simulink model "Copy_of_MPC_control"  (R2018a)
settings: Solver=FixedStepAuto  StartTime=0  StopTime=Tend  FixedStep=0.001  RelTol=5e-3
model workspace (MAT data in the model file):
  A_mu = 10
  B_reff = 8.386
  Cz = 7766.25
  DCT_Param.Transmission.Ratios = [3.78 2.18 1.43 1.03 0.935 0.84]
  DCT_Param.Transmission.Shaft_Inertia_Odd = 0.0023
  DCT_Param.Transmission.Shaft_Inertia_Even = 0.0009
  DCT_Param.Transmission.Shaft_Inertia_Output = 0.008
  DCT_Param.Transmission.Gear_Inertia = 0.001
  DCT_Param.Transmission.Gear_Efficiency = 0.94
  DCT_Param.Transmission.Gear_Ang_Vel_Thr = 0.01
  DCT_Param.Transmission.Shaft_Velocity_Odd = 0
  DCT_Param.Transmission.Shaft_Velocity_Even = 0
  DCT_Param.Transmission.Shaft_Velocity_Output = 0
  DCT_Param.Transmission.Gear_Initial_Velocity = 0
  DCT_Param.Transmission.Abstract.Compliance = 100000
  DCT_Param.Transmission.Abstract.Damping = 10000
  DCT_Param.Transmission.Abstract.Ratio_Time_Const = 0.05
  DCT_Param.Transmission.Abstract.Shift_Gear_Delay = 25
  DCT_Param.Clutch.Torque_Radius = 130
  DCT_Param.Clutch.Num_Friction_Surfaces = 4
  DCT_Param.Clutch.Engagement_Piston_Area = 0.001
  DCT_Param.Clutch.Kinetic_Friction_Coeff = 0.3
  DCT_Param.Clutch.Static_Friction_Coeff = 0.31
  DCT_Param.Clutch.Derating_Factor = 1
  DCT_Param.Clutch.Clutch_Velocity_Tolerance = 0.001
  DCT_Param.Clutch.Threshold_Pressure = 1
  DCT_Param.Clutch.Drag_Torque_Coeff = 0
  DCT_Param.Dog_Clutch.Max_Torque = 1000
  DCT_Param.Dog_Clutch.Teeth_Mean_Radius = 50
  DCT_Param.Dog_Clutch.Tooth_Height = 10
  DCT_Param.Dog_Clutch.Ring_Hub_Clearance = 3
  DCT_Param.Dog_Clutch.Ring_Stop_Stiffness = 1000000
  DCT_Param.Dog_Clutch.Ring_Stop_Damping = 1000
  DCT_Param.Dog_Clutch.Shift_Linkage_Damping = 100
  DCT_Param.Dog_Clutch.Max_Engage_Velocity = 1000000
  DCT_Param.Dog_Clutch.Tooth_Engage_Overlap = 3
  DCT_Param.Vehicle.Mass = 1600
  DCT_Param.Vehicle.Wheels_Per_Axle = 2
  DCT_Param.Vehicle.Distance_CG_FrontAxle = 1.7
  DCT_Param.Vehicle.Distance_CG_RearAxle = 2
  DCT_Param.Vehicle.Distance_CG_Ground = 0.5
  DCT_Param.Vehicle.Frontal_Area = 3
  DCT_Param.Vehicle.Aero_Drag_Coeff = 0.4
  DCT_Param.Vehicle.Initial_Velocity = 0
  DCT_Param.Vehicle.Final_Drive_Ratio = 3.7
  DCT_Param.Vehicle.Final_Drive_Efficiency = 0.86
  DCT_Param.Vehicle.Final_Drive_Vel_Thresh = 0.01
  DCT_Param.Vehicle.Side_Shaft_Inertia = 0.01
  DCT_Param.Vehicle.Side_Shaft_Initial_Velocity = 0
  DCT_Param.Vehicle.Tire.Radius = 0.312
  DCT_Param.Vehicle.Tire.Inertia = 0.5
  DCT_Param.Vehicle.Tire.Initial_Velocity = 0
  DCT_Param.Vehicle.Tire.Slip_Vel_Thresh = 0.1
  DCT_Param.Vehicle.Tire.Nominal_Vertical_Load = 4000
  DCT_Param.Vehicle.Tire.C_Coeff = 1.685
  DCT_Param.Vehicle.Tire.D_Coeff = [1.21 -0.037]
  DCT_Param.Vehicle.Tire.E_Coeff = [0.344 0.095 -0.02 0]
  DCT_Param.Vehicle.Tire.BCD_Coeff = [21.51 -0.163 0.245]
  DCT_Param.Vehicle.Tire.H_Coeff = [-0.002 0.002]
  DCT_Param.Vehicle.Tire.V_Coeff = [0 0]
  DCT_Param.ICE.Max_Power = 100000
  DCT_Param.ICE.Speed_At_Max_Power = 5500
  DCT_Param.ICE.Max_Speed = 7000
  DCT_Param.ICE.Stall_Speed = 200
  DCT_Param.ICE.Shaft_Inertia = 0.2
  DCT_Param.ICE.Initial_Velocity = 800
  DCT_Param.ICE.Idle_Ref_Spd = 800
  DCT_Param.ICE.Engine_Time_Constant = 0.2
  DCT_Param.ICE.Initial_Normalized_Throttle = 0
  DCT_Param.ICE.Speed_Threshold = 20
  DCT_Param.ICE.FC.Speed_Vector = [0 368.421052632 736.842105263 1105.26315789 1473.68421053 1842.10526316 2210.52631579 2578.94736842 2947.36842105 3315.78947368 3684.21052632 4052.63157895 4421.05263158 4789.47368421 5157.89473684 5526.31578947 5894.73684211 6263.15789474 6631.57894737 7000]
  DCT_Param.ICE.FC.Torque_Vector = [0 10.5263157895 21.0526315789 31.5789473684 42.1052631579 52.6315789474 63.1578947368 73.6842105263 84.2105263158 94.7368421053 105.263157895 115.789473684 126.315789474 136.842105263 147.368421053 157.894736842 168.421052632 178.947368421 189.473684211 200]
  DCT_Param.ICE.FC.Consumption_Table = [0.262945178015 0.225304787522 0.201465019624 0.191425874321 0.195187351614 0.212749451502 0.244112173984 0.289275519063 0.348239486736 0.421004077004 0.507569289868 0.607935125326 ... (400 elements, 20x20)]
  DCT_Param.Shift_Map_Example.Pedal_Positions = [0.1 0.4 0.5 0.9]
  DCT_Param.Shift_Map_Example.Upshift_Speeds = [11  20  26  34.5  43; 14  26  35  44.5  55; 17  31  42  52.5  65; 21  39  52  66.5  80]
  DCT_Param.Shift_Map_Example.Downshift_Speeds = [8.9  17  23.6  32.4  40.8; 11.5  22.7  32  41.6  52.2; 14  27  38.1  50  62; 18  33  48  62.6  76.2]
  DCT_Param.Shift_Map_ORIG.Pedal_Positions = [0.1 0.4 0.5 0.9]
  DCT_Param.Shift_Map_ORIG.Upshift_Speeds = [11.5  23.5  35.5  45.5  55.5; 14.5  26.5  38.5  48.5  58.5; 17.5  29.5  41.5  51.5  61.5; 20.5  32.5  44.5  54.5  64.5]
  DCT_Param.Shift_Map_ORIG.Downshift_Speeds = [8.5  20.5  32.5  42.5  52.5; 11.5  23.5  35.5  45.5  55.5; 14.5  26.5  38.5  48.5  58.5; 17.5  29.5  41.5  51.5  61.5]
  DCT_Param.Shift_Map_OPT.Pedal_Positions = [0.1 0.4 0.5 0.9]
  DCT_Param.Shift_Map_OPT.Upshift_Speeds = [17.8469  29.8469  35.8159  41.2981  46.3004; 19.2469  33.9778  43.9778  53.9778  63.9778; 24.5469  41.9778  62.1778  78.5778  106.9778; 27.5469  59.3778  99.0445  109.0445  119.0445]
  DCT_Param.Shift_Map_OPT.Downshift_Speeds = [14.8469  26.8469  32.8159  38.2981  43.3004; 16.2469  30.9778  40.9778  50.9778  60.9778; 21.5469  38.9778  59.1778  75.5778  103.9778; 24.5469  56.3778  96.0445  106.0445  116.0445]
  DCT_Param.Shift_Map.Pedal_Positions = [0.1 0.4 0.5 0.9]
  DCT_Param.Shift_Map.Upshift_Speeds = [11.5  23.5  35.5  45.5  55.5; 14.5  26.5  38.5  48.5  58.5; 17.5  29.5  41.5  51.5  61.5; 20.5  32.5  44.5  54.5  64.5]
  DCT_Param.Shift_Map.Downshift_Speeds = [8.5  20.5  32.5  42.5  52.5; 11.5  23.5  35.5  45.5  55.5; 14.5  26.5  38.5  48.5  58.5; 17.5  29.5  41.5  51.5  61.5]
  DCT_Param.Control.Clutch.Min_Lock_Pressure = 2000000
  DCT_Param.Control.Clutch.Max_Lock_Pressure = 5000000
  DCT_Param.Control.Clutch.Max_Unlock_Pressure = 500000
  DCT_Param.Control.Engine_Start_RPM = 800
  DCT_Param.Control.Engine_Stop_RPM = 790
  DCT_Param.Control.Mode_Logic_TS = 0.1
  DCT_Param.Control.ICE.Kp = 0.02
  DCT_Param.Control.ICE.Ki = 0.01
  DCT_Param.Control.Gen.Kp = 10
  DCT_Param.Control.Gen.Ki = 3
  DCT_Param.Control.Mot.Kp = 500
  DCT_Param.Control.Mot.Ki = 300
  DCT_Param.Control.Veh_Spd.Kp = 0.02
  DCT_Param.Control.Veh_Spd.Ki = 0.04
  DCT_Param.Driver.Kp = 400
  DCT_Param.Driver.Ki = 0.001
  DCT_Param.Driver.Pedal_Filter_Const = 0.01
  DCT_Param.Dog_Clutches.Pulse_Delay = 50
  DCT_Param.Dog_Clutches.Pulse_Length = 20
  DCT_Param.Animation.Teeth_Ratios = [0.338461538462 0.555555555556 0.916666666667 0.96 1.17948717949 1.92307692308]
  DCT_Param.Animation.Teeth_Ratios_Reverse = [0.458333333333 0.75]
  DCT_Param.Shift_Map_OPT506.Pedal_Positions = [0.1 0.4 0.5 0.9]
  DCT_Param.Shift_Map_OPT506.Upshift_Speeds = [18  30.2  48.3  67.3322  77.3429; 20.1  36.85  66.6178  76.7537  86.7537; 21.1  40.25  71.0189  81.0189  91.7873; 24.1  63.75  80.7523  105.9489  115.9489]
  DCT_Param.Shift_Map_OPT506.Downshift_Speeds = [15  27.2  45.3  64.3322  74.3429; 17.1  33.85  63.6178  73.7537  83.7537; 18.1  37.25  68.0189  78.0189  88.7873; 21.1  60.75  77.7523  102.9489  112.9489]
  DCT_Param.Shift_Map_OPTAbsRea176.Pedal_Positions = [0.1 0.4 0.5 0.9]
  DCT_Param.Shift_Map_OPTAbsRea176.Upshift_Speeds = [17.8469  29.8469  35.7875  44.0901  49.4243; 18.9219  34.1312  45.8256  59.7585  69.7585; 32.1719  43.4585  53.51  103.2151  114.6401; 35.1719  59.2585  99.5217  109.5217  119.5217]
  DCT_Param.Shift_Map_OPTAbsRea176.Downshift_Speeds = [14.8469  26.8469  32.7875  41.0901  46.4243; 15.9219  31.1312  42.8256  56.7585  66.7585; 29.1719  40.4585  50.51  100.2151  111.6401; 32.1719  56.2585  96.5217  106.5217  116.5217]
  D_reff = 0.25826
  Downshift_Speeds = [9.5625  23.0625  36.5625  47.8125  59.0625  68.90625  78.75; 12.9375  26.4375  39.9375  51.1875  62.4375  72.84375  83.25; 16.3125  29.8125  43.3125  54.5625  65.8125  76.78125  87.75; 19.6875  33.1875  46.6875  57.9375  69.1875  80.71875  92.25]
  Pedal_Positions = [0.1 0.4 0.5 0.9]
  SUS.Stiffness = 24000
  SUS.Damping.Constant = 1262
  SUS.Damping.Rebound = [4040 4950 2883 2043]
  SUS.Damping.Compression = [3600 3420 1863 1472]
  SUS.PistonSpeed = [0.05 0.1 0.3 0.6]
  SUS.UnsprungMass.Fr = 21.0693333333
  SUS.UnsprungMass.Rr = 21.0693333333
  Upshift_Speeds = [12.9375  26.4375  39.9375  51.1875  62.4375  72.84375  83.25; 16.3125  29.8125  43.3125  54.5625  65.8125  76.78125  87.75; 19.6875  33.1875  46.6875  57.9375  69.1875  80.71875  92.25; 33  52.5  77.25  100.5  138.75  161.875  185]
  VEH.Mass = 1181
  VEH.StaticNormalFrontLoad.FR = 264.666666667
  VEH.StaticNormalFrontLoad.FL = 264.666666667
  VEH.StaticNormalRearLoad.RR = 322
  VEH.StaticNormalRearLoad.RL = 322
  VEH.WheelBase = 3.075
  VEH.FrontAxlePositionfromCG = 1.515
  VEH.RearAxlePositionfromCG = 1.504
  VEH.HeightCG = 0.134
  VEH.FrontalArea = 2.11
  VEH.DragCoefficient = 0.33
  VEH.NumberOfWheelsPerAxle = 2
  VEH.Thread.FR = 1.705
  VEH.Thread.RR = 1.705
  VEH.PitchMomentInertia = 1922.66666667
  VEH.RollMomentInertia = 432.333333333
  VEH.YawMomentInertia = 2066
  VEH.SteeringRatio = 18
  VEH.TrackWidth = 1.922
  VEH.SprungMass = 1096.72266667
  VEH.InitialLongPosition = 0
  VEH.InitialLatPosition = 3.125
  VEH.InitialVertPosition = 0.0111
  VEH.InitialRollAngle = 0
  VEH.InitialPitchAngle = -0.000732
  VEH.InitialYawAngle = 0
  VEH.InitialLongVel = 0
  VEH.InitialLatVel = 0
  VEH.InitialVertVel = 0
  VEH.InitialRollRate = 0
  VEH.InitialPitchRate = 0
  VEH.InitialYawRate = 0
  V_o = 16.7
  V_xlow = 1
  WH.Tire.Radius.Front = 0.384
  WH.Tire.Radius.Rear = 0.401
  WH.Tire.Sidewall = 0.245
  WH.Tire.RollingResistCoeff = 0.0103
  WH.Tire.Magic.B = 10
  WH.Tire.Magic.C = 1.9
  WH.Tire.Magic.D = 1
  WH.Tire.Magic.E = 0.97
  WH.Tire.Magic.Bx = 12
  WH.Tire.Magic.Cx = 1.9
  WH.Tire.Magic.Dx = 0.72
  WH.Tire.Magic.Ex = 0.95
  WH.Tire.Magic.By = 12
  WH.Tire.Magic.Cy = 1.3
  WH.Tire.Magic.Dy = 0.75
  WH.Tire.Magic.Ey = 0.2
  WH.Tire.Front.Ky = 40000
  WH.Tire.Rear.Ky = 40000
  WH.Tire.Kz = 320000
  WH.Tire.Damping = 100
  WH.Inertia = 1.00333333333
  WH.Mass = 11.4333333333
  WH.DampingCoefficient = 0.01
  WH.VelocityTol = 0.1
  a = 1.4
  alpha_max = 1.5
  alpha_min = -1.5
  b = 1.8
  c_zo = 209651
  epsilon = 0.1
  h = 0.134
  path.ISO3888p2.x = [0 2 12 25.5 36.5 49 61]
  path.ISO3888p2.y = [0 0 0 3.725 3.725 0 0]
  path.ISO3888p2.ylb = [1.225 1.225 1.225 4.725 4.725 1.5 1.5]
  path.ISO3888p2.yrb = [-1.225 -1.225 -1.225 2.225 2.225 -1.5 -1.5]
  path.CUSC.x = [10.668 21.336 36.576 54.864 73.152]
  path.CUSC.y = [0 0 5.1816 0 0]
  path.CUSC.ylb = [1.2192 1.2192 7.0104 1.8288 1.8288]
  path.CUSC.yrb = [-1.2192 -1.2192 3.3528 -1.8288 -1.8288]
  pio = 220000
  q_Fcx = 0
  q_Fz2 = 15.4
  q_Fzy = 0
  q_reo = 0.9974
  q_sx1 = -0.007764
  q_sx10 = 0.2824
  q_sx11 = 5.349
  q_sx12 = 0
  q_sx13 = 0
  q_sx14 = 0
  q_sx2 = 1.1915
  q_sx3 = 0.013948
  q_sx4 = 4.912
  q_sx5 = 1.02
  q_sx6 = 22.83
  q_sx7 = 0.7104
  q_sx8 = -0.023393
  q_sx9 = 0.6581
  q_sy1 = 0.00702
  q_sy2 = 0
  q_sy3 = 0.001515
  q_sy4 = 8.514e-05
  q_sy5 = 0
  q_sy6 = 0
  q_sy7 = 0.9008
  q_sy8 = -0.4089
  q_v1 = 0.0007742
  q_v2 = 0.04667
  r_Bx1 = 12.531
  r_Bx2 = 9.532
  r_Bx3 = 0
  r_By1 = 10.615
  r_By2 = 7.705
  r_By3 = 3.433e-06
  r_By4 = 0
  r_Cx1 = 1.019
  r_Cy1 = 1.0585
  r_Ex1 = -0.4487
  r_Ex2 = -0.4726
  r_Ey1 = 0.3132
  r_Ey2 = 7.63e-06
  r_Hx1 = 0.0002374
  r_Hy1 = 0.011646
  r_Hy2 = 7.63e-06
  r_Vy1 = 0.05654
  r_Vy2 = 7.63e-06
  r_Vy3 = 0
  r_Vy4 = 99.9
  r_Vy5 = 2
  r_Vy6 = 15.814
  r_o = 0.3135
  vehWidth = 2
  w = 1
undefined symbols (not defined in the file): C_Brake, C_Final, C_Front, C_Front_1, C_Front_2, C_Middle, C_out_Brake, C_out_Final, C_out_Front, C_out_Front_1, C_out_Front_2, C_out_Middle, Co, Cok_Brake, Cok_Final, Cok_Front_1, Cok_Front_2, Cok_Middle, Cso, D_out_Brake, D_out_Final, D_out_Front, D_out_Front_1, D_out_Front_2, D_out_Middle, Earlytochange, Earlytochange2, F, F_Brake, F_Final, F_Front, F_Front_1, F_Front_2, F_Middle, Fs, G_Brake, G_Final, G_Front_1, G_Front_2, G_Middle, G_sys_Brake, G_sys_Final, G_sys_Front, G_sys_Front_1, G_sys_Front_2, G_sys_Middle, Gd, Gd_Brake, Gd_Final, Gd_Front, Gd_Front_1, Gd_Front_2, Gd_Middle, Go, Gsd, Gso, H_Brake, H_Final, H_Front_1, H_Front_2 ... (+60)
libraries: simulink x10, sim3dlib x4, autolibutils x2, vehdynlibviscommon x2
(part 1 of 8)
settings Model: ModifiedByFormat=The MathWorks, Inc.  Creator=The MathWorks, Inc.  LastModifiedBy=The MathWorks, Inc.
settings SolverCC: ZeroCrossAlgorithm=Adaptive  DecoupledContinuousIntegration=on  MinimalZcImpactIntegration=on
settings DebuggingCC: SignalInfNanChecking=error  ArtificialAlgebraicLoopMsg=none  IgnoredZcDiagnostic=none  ModelReferenceExtraNoncontSigs=none
settings ModelReferenceCC: UpdateModelReferenceTargets=IfOutOfDate  EnableParallelModelReferenceBuilds=on  ModelReferenceMinAlgLoopOccurrences=on  PropagateSignalLabelsOutOfModel=off
settings RTWCC: BuildConfiguration=Faster Runs

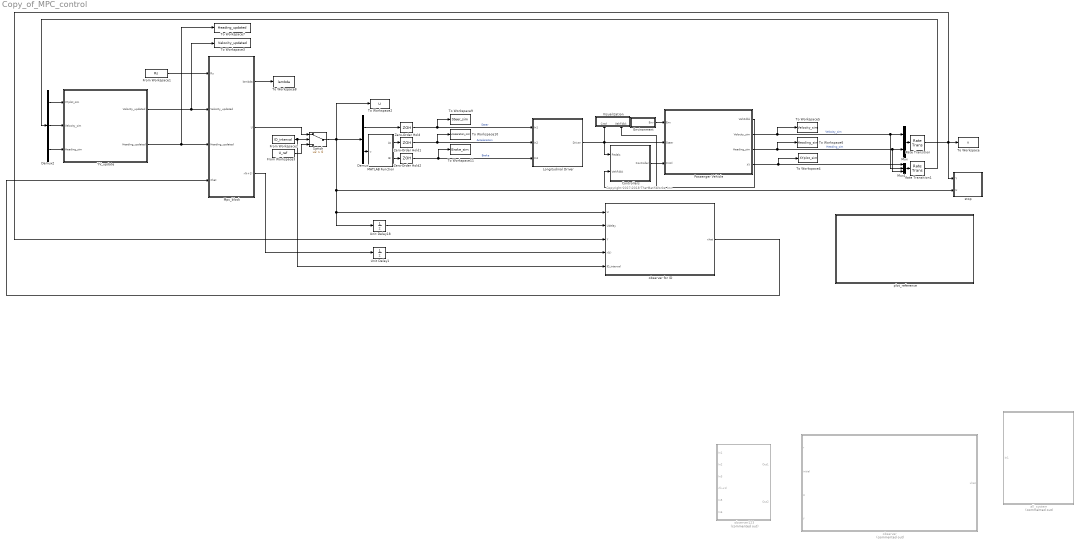
== system Copy_of_MPC_control ==
  note: Copyright 2017-2018 The MathWorks, Inc.
  Controllers : Subsystem
      mask Display: image('SystemControllers.png')
  Demux : Demux  Outputs=2
  Demux2 : Demux  Outputs=3
  Environment : Subsystem  TreatAsAtomicUnit=on
      mask Display: disp('Environment')
  From Workspace1 : FromWorkspace  VariableName=Rs  SampleTime=Ts
  From Workspace2 : FromWorkspace  VariableName=ID_interval  SampleTime=Ts
  From Workspace3 : FromWorkspace  VariableName=U_ref  SampleTime=Ts
  Longitudinal Driver : Subsystem  SystemSampleTime=Tf  VariantControl=0
      mask Display: image('longitudinal_driver_pedals.png');
  MATLAB Function : MATLAB Function  TreatAsAtomicUnit=on  SystemSampleTime=Ts
  Mpc_block : Subsystem  TreatAsAtomicUnit=on  SystemSampleTime=Ts
  Mux : Mux  Inputs=2
  Mux1 : Mux  Inputs=3
  Passenger Vehicle : Subsystem  TreatAsAtomicUnit=on
      settings: MinAlgLoopOccurrences=on
      mask Display: image('PassengerVehicle.png')
  Rate Transition : RateTransition  OutPortSampleTime=Ts
  Rate Transition1 : RateTransition  OutPortSampleTime=Ts
  Switch : Switch  Criteria=u2 > Threshold
  To Workspace : ToWorkspace  VariableName=Y  SampleTime=Ts
  To Workspace10 : ToWorkspace  VariableName=Acceleration_sim  SampleTime=Tf
  To Workspace11 : ToWorkspace  VariableName=Brake_sim  SampleTime=Tf
  To Workspace2 : ToWorkspace  VariableName=U  SampleTime=Ts
  To Workspace3 : ToWorkspace  VariableName=Velocity_updated  SampleTime=Ts
      settings: Save2DSignal=2-D array (concatenate along first dimension)
  To Workspace4 : ToWorkspace  VariableName=XYplot_sim  SampleTime=Ts
  To Workspace5 : ToWorkspace  VariableName=Velocity_sim  SampleTime=Ts
  To Workspace6 : ToWorkspace  VariableName=Heading_sim  SampleTime=Ts
  To Workspace7 : ToWorkspace  VariableName=Heading_updated  SampleTime=Ts
      settings: Save2DSignal=2-D array (concatenate along first dimension)
  To Workspace8 : ToWorkspace  VariableName=lambda  SampleTime=Ts
  To Workspace9 : ToWorkspace  VariableName=Steer_sim  SampleTime=-1
  Unit Delay1 : UnitDelay  InitialCondition=ro  SampleTime=Ts
  Unit Delay18 : UnitDelay  InitialCondition=[0;0]  SampleTime=Ts
  Visualization : Subsystem  TreatAsAtomicUnit=on
      mask Display: disp('Visualization')
  YV_update : Subsystem  TreatAsAtomicUnit=on
  Zero-Order Hold : ZeroOrderHold  SampleTime=Tf
  Zero-Order Hold1 : ZeroOrderHold  SampleTime=Tf
  Zero-Order Hold2 : ZeroOrderHold  SampleTime=Tf
  all_system : Subsystem  Commented=on
  observer : Subsystem  Commented=on
  observer for ID : Subsystem
  observer123 : Subsystem  Commented=on
  plot_reference : Subsystem
      settings: MinAlgLoopOccurrences=on
  stop : Subsystem
  wires:
  Longitudinal Driver/1(Driver) -> Passenger Vehicle/2(Steer), Controllers/1(Pedals), Visualization/1(Cntrl)
  Environment/1(Env) -> Passenger Vehicle/1(Env)
  Controllers/1(Controller) -> Passenger Vehicle/3(Cntrl)
  Passenger Vehicle/1(VehFdbk) -> Controllers/2(VehFdbk), Visualization/2(VehFdbk)
  Demux/1 -> Zero-Order Hold/1
  MATLAB Function/1(Ac) -> Zero-Order Hold1/1
  MATLAB Function/2(Br) -> Zero-Order Hold2/1
  Passenger Vehicle/3(Heading_sim) -> To Workspace6/1, Mux/2, Mux1/3  "Heading_sim"
  Mux/1 -> Rate Transition/1
  Demux/2 -> MATLAB Function/1(u)
  Zero-Order Hold/1 -> To Workspace9/1, Longitudinal Driver/1(In1)  "Steer"
  Zero-Order Hold1/1 -> To Workspace10/1, Longitudinal Driver/2(In2)  "Acceleration"
  Zero-Order Hold2/1 -> To Workspace11/1, Longitudinal Driver/3(In3)  "Brake"
  Passenger Vehicle/2(Velocity_sim) -> To Workspace5/1, Mux/1, Mux1/2  "Velocity_sim"
  YV_update/2(Heading_updated) -> Mpc_block/3(Heading_updated), To Workspace7/1
  YV_update/1(Velocity_updated) -> Mpc_block/2(Velocity_updated), To Workspace3/1
  Demux2/2 -> YV_update/2(Velocity_sim)
  Mux1/1 -> Rate Transition1/1
  Demux2/1 -> YV_update/1(XYplot_sim)
  Demux2/3 -> YV_update/3(Heading_sim)
  Rate Transition1/1 -> Demux2/1
  From Workspace1/1 -> Mpc_block/1(Rs)
  Passenger Vehicle/4(XY) -> To Workspace4/1, Mux1/1
  observer for ID/1(xhat) -> Mpc_block/4(Xhat)
  Rate Transition/1 -> observer for ID/3(Y), To Workspace/1, stop/1(Y)
  Mpc_block/3(r(k+1)) -> Unit Delay1/1
  Mpc_block/1(lambda) -> To Workspace8/1
  From Workspace2/1 -> observer for ID/5(ID_interval), Switch/2
  Mpc_block/2(U) -> Switch/1
  Switch/1 -> Demux/1, Unit Delay18/1, observer for ID/1(U), stop/2(U), To Workspace2/1
  From Workspace3/1 -> Switch/3
  Unit Delay18/1 -> observer for ID/2(Udelay)
  Unit Delay1/1 -> observer for ID/4(r(k))

== system Copy_of_MPC_control/Controllers ==
  Pedals : Inport
  VehFdbk : Inport  Port=2
  Brake Controller : Subsystem
  Bus Creator : BusCreator  Inputs=1
  Bus Creator1 : BusCreator  Inputs=1
  Bus Creator2 : BusCreator  Inputs=1
  Bus Creator3 : BusCreator  Inputs=3
  Bus Selector : BusSelector  OutputSignals=Body.xdot,Wheels.kappa
  Bus Selector1 : BusSelector  OutputSignals=Driveline.EngSpd,Driveline.PropShftSpd
  Bus Selector2 : BusSelector  OutputSignals=Accel,Brake
  ECU : Subsystem
  Transmission Controller : Subsystem
  Controller : Outport
  wires:
  Transmission Controller/1(Gear) -> Bus Creator1/1  "GearCmd"
  Bus Selector/2 -> Brake Controller/3(kappa)  "<kappa>"
  ECU/1(Trq Cmd) -> Bus Creator/1  "EngTrqCmd"
  Brake Controller/1(PCmd) -> Bus Creator2/1  "PrsCmd"
  VehFdbk/1 -> Bus Selector/1, Bus Selector1/1
  Bus Selector/1 -> Brake Controller/2(xdot)  "<xdot>"
  Bus Selector1/1 -> Transmission Controller/2(EngSpd)  "<EngSpd>"
  Bus Selector1/2 -> Transmission Controller/3(PropShaftSpd)  "<PropShftSpd>"
  Pedals/1 -> Bus Selector2/1
  Bus Selector2/1 -> Transmission Controller/1(Acc), ECU/1(<Accel>)  "<Accel>"
  Bus Selector2/2 -> Brake Controller/1(BrkPrsCmd)  "<Brake>"
  Bus Creator/1 -> Bus Creator3/1  "ECU"
  Bus Creator1/1 -> Bus Creator3/2  "Transmission"
  Bus Creator2/1 -> Bus Creator3/3  "Brake"
  Bus Creator3/1 -> Controller/1  "Controller"

== system Copy_of_MPC_control/Environment ==
  Bus Creator : BusCreator  Inputs=4
  Bus Creator1 : BusCreator  Inputs=2
  Bus Creator2 : BusCreator  Inputs=4
  Bus Creator3 : BusCreator  Inputs=2
  Constant1 : Constant  Value=zeros(4,1)
  Constant3 : Constant  Value=0
  Constant4 : Constant  Value=0
  Constant5 : Constant  Value=0
  Demux : Demux
  Demux1 : Demux
  Friction : Constant  Value=ones(4,1).*1
  Vector Concatenate : Concatenate  NumInputs=3
  Env : Outport
  wires:
  Constant1/1 -> Demux/1
  Bus Creator2/1 -> Bus Creator3/2  "mu"
  Bus Creator/1 -> Bus Creator3/1  "z"
  Demux/2 -> Bus Creator/2  "G_FR_z"
  Demux/3 -> Bus Creator/3  "G_RL_z"
  Constant5/1 -> Vector Concatenate/3  "Z"
  Demux/1 -> Bus Creator/1  "G_FL_z"
  Vector Concatenate/1 -> Bus Creator1/1  "Wind"
  Constant3/1 -> Vector Concatenate/1  "X"
  Demux/4 -> Bus Creator/4  "G_RR_z"
  Constant4/1 -> Vector Concatenate/2  "Y"
  Demux1/3 -> Bus Creator2/3  "mu_RL"
  Demux1/4 -> Bus Creator2/4  "mu_RR"
  Demux1/2 -> Bus Creator2/2  "mu_FR"
  Demux1/1 -> Bus Creator2/1  "mu_FL"
  Friction/1 -> Demux1/1
  Bus Creator3/1 -> Bus Creator1/2  "Gnd"
  Bus Creator1/1 -> Env/1

== system Copy_of_MPC_control/Longitudinal Driver ==
  In1 : Inport  SampleTime=Tf
  In2 : Inport  Port=2  SampleTime=Tf
  In3 : Inport  Port=3  SampleTime=Tf
  Bus Creator1 : BusCreator  Inputs=3
  Driver : Outport
  wires:
  Bus Creator1/1 -> Driver/1
  In2/1 -> Bus Creator1/2  "Accel"
  In3/1 -> Bus Creator1/3  "Brake"
  In1/1 -> Bus Creator1/1  "Steer"

== system Copy_of_MPC_control/Mpc_block ==
  Rs : Inport  SampleTime=Ts  LockScale=on
  Velocity_updated : Inport  Port=2  SampleTime=Ts
  Heading_updated : Inport  Port=3  SampleTime=Ts  LockScale=on
  Xhat : Inport  Port=4
  Constant1 : Constant  Value=M  VectorParams1D=off  SampleTime=-1
  Constant16 : Constant  Value=U_max  VectorParams1D=off  SampleTime=-1
  Constant2 : Constant  Value=Np  SampleTime=-1
  Constant4 : Constant  Value=U_min  VectorParams1D=off  SampleTime=-1
  Constant5 : Constant  Value=JF_part  VectorParams1D=off  SampleTime=-1
  Constant6 : Constant  Value=JE  VectorParams1D=off  SampleTime=-1
  Digital Clock : DigitalClock  SampleTime=Ts
  F : Gain  Gain=F  Multiplication=Matrix(K*u) (u vector)
  Mpc : MATLAB Function  TreatAsAtomicUnit=on  SystemSampleTime=Ts
  Unit Delay : UnitDelay  InitialCondition=[0;0]  SampleTime=Ts
  lambda : Outport
  U : Outport  Port=2
  r(k+1) : Outport  Port=3
  wires:
  Unit Delay/1 -> Mpc/12(U_delay)
  Heading_updated/1 -> Mpc/8(Heading_updated)
  Constant1/1 -> Mpc/4(M)
  Mpc/3(U) -> U/1, Unit Delay/1
  Constant2/1 -> Mpc/5(Np)
  Xhat/1 -> F/1
  Rs/1 -> Mpc/10(Rs)
  Constant4/1 -> Mpc/6(U_min)
  Velocity_updated/1 -> Mpc/9(Velocity_updated)
  Constant6/1 -> Mpc/1(JE)
  Mpc/2(r) -> r(k+1)/1
  Digital Clock/1 -> Mpc/11(Tsim)
  Constant16/1 -> Mpc/7(U_max)
  Mpc/1(lambda) -> lambda/1
  F/1 -> Mpc/3(Fxh)
  Constant5/1 -> Mpc/2(JF_part)

== system Copy_of_MPC_control/Passenger Vehicle ==
  Env : Inport
  Steer : Inport  Port=2
  Cntrl : Inport  Port=3
  "Body, Suspension, Wheels" : Subsystem  Variant=on  OverrideUsingVariant=1
  Bus Creator2 : BusCreator  Inputs=4
  Engine : Subsystem  Variant=on  OverrideUsingVariant=0
  Mux : Mux  Inputs=2
  "Steering, Transmission, Driveline and Brakes" : Subsystem  Variant=on  OverrideUsingVariant=0
  Subsystem : Subsystem
  Subsystem1 : Subsystem
  Subsystem2 : Subsystem
  Subsystem3 : Subsystem
  Subsystem4 : Subsystem
  Subsystem5 : Subsystem
  Sum1 : Sum
  To Workspace1 : ToWorkspace  VariableName=Vy_sim  SampleTime=Ts
  To Workspace2 : ToWorkspace  VariableName=Vx_sim  SampleTime=Ts
  To Workspace3 : ToWorkspace  VariableName=Beta_sim  SampleTime=Ts
  beta : MATLAB Function  TreatAsAtomicUnit=on  SystemSampleTime=Tf
      settings: MinAlgLoopOccurrences=on
  VehFdbk : Outport
  Velocity_sim : Outport  Port=2
  Heading_sim : Outport  Port=3
  XY : Outport  Port=4
  wires:
  Bus Creator2/1 -> VehFdbk/1
  Env/1 -> Subsystem/1(Env)
  Subsystem1/1(Driveline) -> [Driveline], Bus Creator2/2  "Driveline"
  "Steering, Transmission, Driveline and Brakes"/1(WhlAng) -> Subsystem1/1(WhlAng)
  "Steering, Transmission, Driveline and Brakes"/2(AxlTrq) -> Subsystem1/2(AxlTrq)
  "Steering, Transmission, Driveline and Brakes"/3(BrkPrs) -> Subsystem1/3(BrkPrs)
  "Steering, Transmission, Driveline and Brakes"/4(EngSpd) -> Subsystem1/4(EngSpd)
  "Steering, Transmission, Driveline and Brakes"/5(PropShftSpd) -> Subsystem1/5(PropShftSpd)
  Steer/1 -> Subsystem2/2(SteerCmd)
  Cntrl/1 -> Subsystem3/1(Cntrl), Subsystem2/1(Cntrl)
  Subsystem2/1(Steer) -> "Steering, Transmission, Driveline and Brakes"/1(SteerHWCmd)
  Subsystem2/3(GearCmd) -> "Steering, Transmission, Driveline and Brakes"/3(GearCmd)
  Subsystem2/4(PrsCmd) -> "Steering, Transmission, Driveline and Brakes"/4(BrkPrsCmd)
  Subsystem2/5(omega) -> "Steering, Transmission, Driveline and Brakes"/5(omega)
  Engine/1(EngTrq) -> Subsystem5/1("EngTrq ")
  Subsystem2/2(EngTrq) -> "Steering, Transmission, Driveline and Brakes"/2(EngTrq)
  Subsystem3/1(EngTrqCmd) -> Engine/1(TrqCmd)
  Subsystem3/2(EngSpd) -> Engine/2(EngSpd)
  Subsystem4/1(Chassis) -> Bus Creator2/3  "Body"
  Subsystem4/2(Wheels) -> Bus Creator2/4, [Wheels]  "Wheels"
  Subsystem5/1(Eng) -> [EngTrq], Bus Creator2/1  "Engine"
  [Driveline] -> Subsystem/2(Driveline)
  [Wheels] -> Subsystem2/4(Wheels)
  [EngTrq] -> Subsystem2/3(EngTrqCmd)
  [Driveline] -> Subsystem3/2(Driveline)
  "Body, Suspension, Wheels"/19(XWheel) -> Subsystem4/19(XWheel)
  "Body, Suspension, Wheels"/11(p) -> Subsystem4/11(p)
  "Body, Suspension, Wheels"/12(q) -> Subsystem4/12(q)
  "Body, Suspension, Wheels"/7(Ydot) -> Subsystem4/7(Ydot)
  "Body, Suspension, Wheels"/13(r) -> Subsystem4/13(r)
  "Body, Suspension, Wheels"/16(zAxle) -> Subsystem4/16(zAxle)
  "Body, Suspension, Wheels"/8(phi) -> Subsystem4/8(phi)
  "Body, Suspension, Wheels"/3(X) -> Mux/1, Subsystem4/3(X)
  Subsystem/6(BrkPrs) -> "Body, Suspension, Wheels"/6(BrkPrs)
  "Body, Suspension, Wheels"/9(theta) -> Subsystem4/9(theta)
  "Body, Suspension, Wheels"/5(Z) -> Subsystem4/5(Z)
  Subsystem/3(mu) -> "Body, Suspension, Wheels"/3(Friction)
  "Body, Suspension, Wheels"/17(omega) -> Subsystem4/17(omega)
  Subsystem/4(WhlAng) -> "Body, Suspension, Wheels"/4(WheelAngle)
  "Body, Suspension, Wheels"/14(ay) -> Subsystem4/14(ay)
  Subsystem/1(Wind) -> "Body, Suspension, Wheels"/1(WindXYZ)
  Subsystem/2(Gnd) -> "Body, Suspension, Wheels"/2(Ground)
  "Body, Suspension, Wheels"/10(psi) -> Subsystem4/10(psi), Sum1/2
  "Body, Suspension, Wheels"/4(Y) -> Mux/2, Subsystem4/4(Y)
  Subsystem/5(AxleTrq) -> "Body, Suspension, Wheels"/5(AxleTrq)
  "Body, Suspension, Wheels"/18(ZHP) -> Subsystem4/18(ZHP)
  "Body, Suspension, Wheels"/20(YWheel) -> Subsystem4/20(YWheel)
  "Body, Suspension, Wheels"/6(Xdot) -> Subsystem4/6(Xdot)
  "Body, Suspension, Wheels"/15(kappa) -> Subsystem4/15(kappa)
  Mux/1 -> XY/1
  Sum1/1 -> Heading_sim/1
  beta/1(beta) -> To Workspace3/1, Sum1/1
  "Body, Suspension, Wheels"/2(ydot) -> To Workspace1/1, beta/2(ydot), Subsystem4/2(ydot)
  "Body, Suspension, Wheels"/1(xdot) -> To Workspace2/1, beta/1(xdot), Subsystem4/1(xdot)
  beta/2(Velocity) -> Velocity_sim/1

== system Copy_of_MPC_control/Visualization ==
  note: Driver Commands
  note: Vehicle Response
  Cntrl : Inport
  VehFdbk : Inport  Port=2
  3D Engine : Subsystem  Variant=on  OverrideUsingVariant=0  mask(3D Engine){engine3D=Disabled, SceneDesc=Straight road, dt3D=.03}
      mask prompts: engine3D "3D Engine"; SceneDesc "Scene Description:"; dt3D "Engine frame rate, dt3D [s]:"
      mask help: This subsystem contains the interface blocks which permit the display of the vehicle in 3D virtual environment. Enable it to view the simulation progress, disable it to inhibit the display.
      mask init:
      | switch get_param(gcb,'engine3D')
      |     case 'Disabled'
      |         set_param(gcb,'OverrideUsingVariant','0')
      |     case 'Enabled'
      |        set_param(gcb,'OverrideUsingVariant','1')
      |     otherwise
      |        set_param(gcb,'OverrideUsingVariant','0')
      | end
      settings: AttributesFormatString=%<engine3D>
      mask Help: eval('vdynblkshelp(''vdynblksscenecameraray'')');
      mask TypeOptions engine3D: Enabled | Disabled
      mask Callback engine3D:
      | switch get_param(gcb,'engine3D')
      |     case 'Disabled'
      |         set_param(gcb,'OverrideUsingVariant','0')
      |     case 'Enabled'
      |        set_param(gcb,'OverrideUsingVariant','1')
      |     otherwise
      |        set_param(gcb,'OverrideUsingVariant','0')
      | end
      mask TypeOptions SceneDesc:
      | 3D Engine/Simulation 3D Engine
      | 1/SceneDesc
      mask Display: disp('3D Engine')
  Acceleration Cmd : Subsystem  DialogController=hmiCreateDDGDialog  IsWebBlock=on  mask(MWDashboardBlock){webBlockId=2ec56b20-76c2-4aac-ab3d-2dd24ca42fe8, webBlockType=lineargauge, ShowInLibBrowser=on, ShowInitialText=on, HMISrcModelName=[]}
      mask prompts: webBlockId "WebBlock Id"; webBlockType "WebBlock Type"; HMISrcModelName "Source Model"
      mask help: SimulinkHMI:dialogs:LinearGaugeDialogDesc
      mask Help: helpview([docroot '/mapfiles/simulink.map'], 'hmi_linear_gauge')
      mask Display:
      | if strcmp(get_param(bdroot(gcb),'BlockDiagramType'), 'library')
      |     image([(matlabroot) '/toolbox/simulink/hmi/icons/LinearGauge.png']);
      | end
  Brake Cmd : Subsystem  DialogController=hmiCreateDDGDialog  IsWebBlock=on  mask(MWDashboardBlock){webBlockId=d9917a9d-f04e-4f5f-9d8a-619b2f9adbbc, webBlockType=lineargauge, ShowInLibBrowser=on, ShowInitialText=on, HMISrcModelName=[]}
      mask prompts: webBlockId "WebBlock Id"; webBlockType "WebBlock Type"; HMISrcModelName "Source Model"
      mask help: SimulinkHMI:dialogs:LinearGaugeDialogDesc
      mask Help: helpview([docroot '/mapfiles/simulink.map'], 'hmi_linear_gauge')
      mask Display:
      | if strcmp(get_param(bdroot(gcb),'BlockDiagramType'), 'library')
      |     image([(matlabroot) '/toolbox/simulink/hmi/icons/LinearGauge.png']);
      | end
  Bus Selector : BusSelector  OutputSignals=Driveline.EngSpd,Body.xdot,Body.ay
  Bus Selector2 : BusSelector  OutputSignals=Accel,Brake,Steer
  Bus Selector3 : BusSelector  OutputSignals=Body.r
  Engine Tach [rpm] : Subsystem  DialogController=hmiCreateDDGDialog  IsWebBlock=on  mask(MWDashboardBlock){webBlockId=b43bb858-1bc3-4216-8222-68d06605e534, webBlockType=circulargauge, ShowInLibBrowser=on, ShowInitialText=on, HMISrcModelName=[]}
      mask prompts: webBlockId "WebBlock Id"; webBlockType "WebBlock Type"; HMISrcModelName "Source Model"
      mask help: SimulinkHMI:dialogs:CircularGaugeDialogDesc
      mask Help: helpview([docroot '/mapfiles/simulink.map'], 'hmi_gauge')
      mask Display:
      | if strcmp(get_param(bdroot(gcb),'BlockDiagramType'), 'library')
      |     image([(matlabroot) '/toolbox/simulink/hmi/icons/CircularGauge.png']);
      | end
  Handwheel Angle [deg] : Subsystem  DialogController=hmiCreateDDGDialog  IsWebBlock=on  mask(MWDashboardBlock){webBlockId=4efaf655-7637-4550-9856-9a687d94287b, webBlockType=semicirculargauge, ShowInLibBrowser=on, ShowInitialText=on, HMISrcModelName=[]}
      mask prompts: webBlockId "WebBlock Id"; webBlockType "WebBlock Type"; HMISrcModelName "Source Model"
      mask help: SimulinkHMI:dialogs:SemicircularGaugeDialogDesc
      mask Help: helpview([docroot '/mapfiles/simulink.map'], 'hmi_half_gauge')
      mask Display:
      | if strcmp(get_param(bdroot(gcb),'BlockDiagramType'), 'library')
      |     image([(matlabroot) '/toolbox/simulink/hmi/icons/SemicircularGauge.png']);
      | end
  Lateral Acceleration [g] : Subsystem  DialogController=hmiCreateDDGDialog  IsWebBlock=on  mask(MWDashboardBlock){webBlockId=4c84f06f-3c50-4c9f-a814-1d904b0076de, webBlockType=semicirculargauge, ShowInLibBrowser=on, ShowInitialText=on, HMISrcModelName=[]}
      mask prompts: webBlockId "WebBlock Id"; webBlockType "WebBlock Type"; HMISrcModelName "Source Model"
      mask help: SimulinkHMI:dialogs:SemicircularGaugeDialogDesc
      mask Help: helpview([docroot '/mapfiles/simulink.map'], 'hmi_half_gauge')
      mask Display:
      | if strcmp(get_param(bdroot(gcb),'BlockDiagramType'), 'library')
      |     image([(matlabroot) '/toolbox/simulink/hmi/icons/SemicircularGauge.png']);
      | end
  Rate Transition1 : RateTransition
  Rate Transition2 : RateTransition
  Signal Specification : SignalSpecification  Unit=deg
  Signal Specification1 : SignalSpecification  Unit=mph
  Signal Specification2 : SignalSpecification  Unit=deg/s
  Signal Specification3 : SignalSpecification  Unit=rpm
  Speed [mph] : Subsystem  DialogController=hmiCreateDDGDialog  IsWebBlock=on  mask(MWDashboardBlock){webBlockId=6d425e54-616c-4430-b762-4652b407af79, webBlockType=circulargauge, ShowInLibBrowser=on, ShowInitialText=on, HMISrcModelName=[]}
      mask prompts: webBlockId "WebBlock Id"; webBlockType "WebBlock Type"; HMISrcModelName "Source Model"
      mask help: SimulinkHMI:dialogs:CircularGaugeDialogDesc
      mask Help: helpview([docroot '/mapfiles/simulink.map'], 'hmi_gauge')
      mask Display:
      | if strcmp(get_param(bdroot(gcb),'BlockDiagramType'), 'library')
      |     image([(matlabroot) '/toolbox/simulink/hmi/icons/CircularGauge.png']);
      | end
  Start Steering Command : LampBlock  WebBlockId=3552  LabelPosition=Hide
  Steer vs Ay : simulink/Sinks/XY Graph  Commented=on  xmin=-300  xmax=300  ymin=-1.5  ymax=1.5  st=.1
  "Steer, Velocity, Lat Accel" : Scope  NumInputPorts=3
  Terminator{,1..3} (4 alike) : Terminator
  Unit Conversion{1..4} (4 alike) : UnitConversion
  Vehicle XY Plotter : Subsystem  mask(Vehicle XY Plotter){a=VEH.FrontAxlePositionfromCG, b=VEH.RearAxlePositionfromCG, w=VEH.TrackWidth, bufferSize=1024, pltDT=0.1}
      mask prompts: a "Distance to front axle from CG, a [m]:"; b "Distance to rear axle from CG, b [m]:"; w "Track width, w [m]:"; bufferSize "Path buffer sampe size, bufferSize []:"; pltDT "Plot update rate, pltDT [s]:"
      mask help: This block will display a MATLAB figure which indicates the vehicle path, current position and heading velocity.
      mask TypeOptions a: Vehicle XY Plotter/a
      mask TypeOptions b: Vehicle XY Plotter/b
      mask TypeOptions w: Vehicle XY Plotter/w
      mask TypeOptions bufferSize: Vehicle XY Plotter/bufferSize
  Yaw Rate and Steer : Scope  NumInputPorts=2
  wires:
  Unit Conversion3/1 -> Signal Specification2/1
  Bus Selector3/1 -> Unit Conversion3/1  "<r>"
  Signal Specification2/1 -> Yaw Rate and Steer/1
  Unit Conversion4/1 -> Signal Specification3/1
  Signal Specification3/1 -> Terminator3/1  "Engine_rpm"
  Signal Specification/1 -> Yaw Rate and Steer/2, Rate Transition1/1, "Steer, Velocity, Lat Accel"/1  "SteerAngle"
  Bus Selector2/3 -> Unit Conversion2/1  "<Steer>"
  Signal Specification1/1 -> Terminator/1  "xdot_mph"
  Unit Conversion1/1 -> Signal Specification1/1
  Bus Selector/3 -> Rate Transition2/1, "Steer, Velocity, Lat Accel"/3  "<ay>"
  Bus Selector2/1 -> Terminator1/1  "<Accel>"
  Rate Transition1/1 -> Steer vs Ay/1
  Unit Conversion2/1 -> Signal Specification/1
  Bus Selector/2 -> "Steer, Velocity, Lat Accel"/2, Unit Conversion1/1  "<xdot>"
  VehFdbk/1 -> Bus Selector3/1, Bus Selector/1, Vehicle XY Plotter/1(VehFdbk), 3D Engine/1(VehFdbk)  "VehFdbk"
  Cntrl/1 -> Bus Selector2/1
  Rate Transition2/1 -> Steer vs Ay/2
  Bus Selector/1 -> Unit Conversion4/1  "<EngSpd>"
  Bus Selector2/2 -> Terminator2/1  "<Brake>"

== system Copy_of_MPC_control/YV_update ==
  XYplot_sim : Inport
  Velocity_sim : Inport  Port=2
  Heading_sim : Inport  Port=3
  Constant2 : Constant  Value=Ts  SampleTime=Ts
  From Workspace1 : FromWorkspace  VariableName=Tsim  SampleTime=Ts
  From Workspace3 : FromWorkspace  VariableName=XYplot_ref  SampleTime=Ts
  MATLAB Function2 : MATLAB Function  TreatAsAtomicUnit=on  SystemSampleTime=Ts
  Velocity_updated : Outport
  Heading_updated : Outport  Port=2
  wires:
  MATLAB Function2/1(Velocity_updated) -> Velocity_updated/1
  From Workspace3/1 -> MATLAB Function2/1(XYplot_ref)
  MATLAB Function2/2(Heading_updated) -> Heading_updated/1
  From Workspace1/1 -> MATLAB Function2/6(Tsim)
  XYplot_sim/1 -> MATLAB Function2/2(XYplot_sim)
  Velocity_sim/1 -> MATLAB Function2/3(Velocity_sim)
  Heading_sim/1 -> MATLAB Function2/4(Yaw_sim)
  Constant2/1 -> MATLAB Function2/5(Ts)

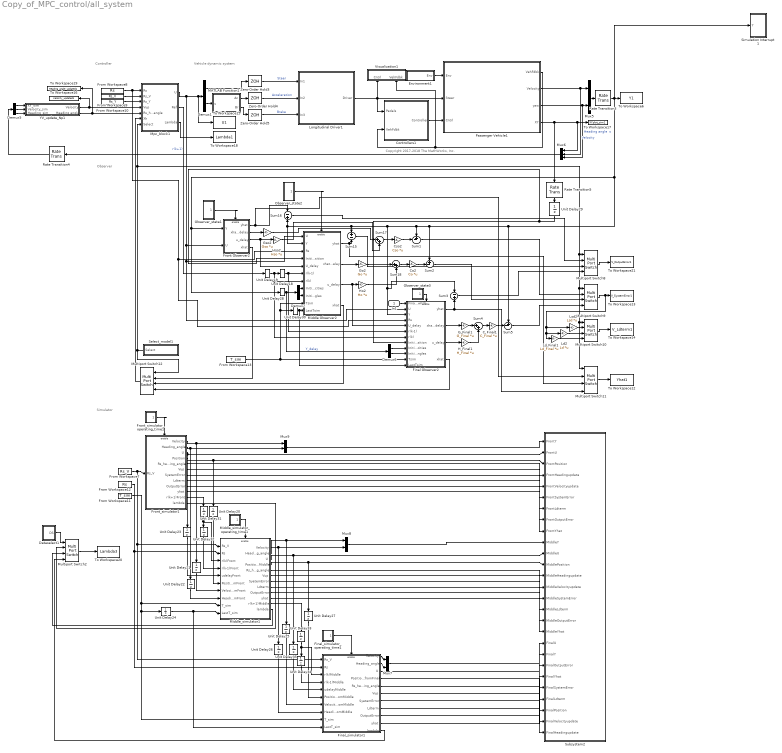
== system Copy_of_MPC_control/all_system ==
  note: Copyright 2017-2018 The MathWorks, Inc.
  note: Controller
  note: Vehicle dynamic system
  note: Observer
  note: Simulator
  In1 : Inport
  C_Final1 : Gain  Gain=C_Final  Multiplication=Matrix(K*u) (u vector)
  Co2 : Gain  Gain=Co  Multiplication=Matrix(K*u) (u vector)
  Controllers1 : Subsystem
      mask Display: image('SystemControllers.png')
  Cso2 : Gain  Gain=Cso  Multiplication=Matrix(K*u) (u vector)
  Dataselect1 : Subsystem
  Demux1 : Demux  Outputs=2
  Demux5 : Demux  Outputs=3
  Demux6 : Demux  Outputs=2
  Demux7 : Demux  Outputs=2
  Environment1 : Subsystem  TreatAsAtomicUnit=on
      mask Display: disp('Environment')
  Final Observer2 : Subsystem
  Final_simulator1 : Subsystem
  Final_simulator_ operating_time1 : Subsystem
  From Workspace10 : FromWorkspace  VariableName=Rs_Y  SampleTime=Ts
  From Workspace11 : FromWorkspace  VariableName=T_sim  SampleTime=Ts
  From Workspace12 : FromWorkspace  VariableName=Rs  SampleTime=Ts
  From Workspace13 : FromWorkspace  VariableName=T_sim  SampleTime=Ts
  From Workspace7 : FromWorkspace  VariableName=Rs_V  SampleTime=Ts
  From Workspace8 : FromWorkspace  VariableName=Rs  SampleTime=Ts
  From Workspace9 : FromWorkspace  VariableName=Rs_V  SampleTime=Ts
  Front Observer2 : Subsystem
  Front_simulator1 : Subsystem
  Front_simulator_ operating_time1 : Subsystem
  G_Final1 : Gain  Gain=G_Final  Multiplication=Matrix(K*u) (u vector)
  Go2 : Gain  Gain=Go  Multiplication=Matrix(K*u) (u vector)
  Gso2 : Gain  Gain=Gso  Multiplication=Matrix(K*u) (u vector)
  H_Final1 : Gain  Gain=H_Final  Multiplication=Matrix(K*u) (u vector)
  Ho2 : Gain  Gain=Ho  Multiplication=Matrix(K*u) (u vector)
  Hso2 : Gain  Gain=Hso  Multiplication=Matrix(K*u) (u vector)
  Ld2 : Gain  Gain=Ld  Multiplication=Matrix(K*u) (u vector)
  Ld_Final1 : Gain  Gain=Ld_Final  Multiplication=Matrix(K*u) (u vector)
  Longitudinal Driver1 : Subsystem  SystemSampleTime=Tf  VariantControl=0
      mask Display: image('longitudinal_driver_pedals.png');
  Lsd2 : Gain  Gain=Lsd  Multiplication=Matrix(K*u) (u vector)
  MATLAB Function1 : MATLAB Function  TreatAsAtomicUnit=on  SystemSampleTime=Ts
  Middle Observer2 : Subsystem
  Middle_simulator1 : Subsystem
  Middle_simulator_ operating_time1 : Subsystem
  Mpc_block1 : Subsystem  TreatAsAtomicUnit=on  SystemSampleTime=Ts
  Multiport Switch{2,8..12} (6 alike) : MultiPortSwitch
  Mux{5,7..9} (4 alike) : Mux  Inputs=2
  Mux6 : Mux  Inputs=3
  Observer_state1 : Subsystem
  Observer_state2 : Subsystem
  Observer_state3 : Subsystem
  Passenger Vehicle1 : Subsystem  TreatAsAtomicUnit=on
      settings: MinAlgLoopOccurrences=on
      mask Display: image('PassengerVehicle.png')
  Rate Transition3 : RateTransition  OutPortSampleTime=Ts
  Rate Transition4 : RateTransition  OutPortSampleTime=Ts
  Rate Transition5 : RateTransition  OutPortSampleTime=Ts
  Select_model1 : Subsystem
  Simulation Interrupt 1 : Subsystem
  Subsystem2 : Subsystem
  Sum1 : Sum  Inputs=+-|
  Sum15 : Sum  Inputs=+-
  Sum16 : Sum  Inputs=-+
  Sum17 : Sum  Inputs=|++
  Sum18 : Sum  Inputs=|++
  Sum2 : Sum  Inputs=+-|
  Sum3 : Sum  Inputs=-+
  Sum4 : Sum  Inputs=|++
  Sum5 : Sum  Inputs=+-|
  To Workspace12 : ToWorkspace  VariableName=Yhat1  SampleTime=Ts
  To Workspace13 : ToWorkspace  VariableName=V_SystemError1  SampleTime=Ts
  To Workspace14 : ToWorkspace  VariableName=V_Ldterm1  SampleTime=Ts
  To Workspace15 : ToWorkspace  VariableName=U1  SampleTime=Ts
  To Workspace16 : ToWorkspace  VariableName=Velocity_updated1  SampleTime=Ts
      settings: Save2DSignal=2-D array (concatenate along first dimension)
  To Workspace17 : ToWorkspace  VariableName=XYplot_sim1  SampleTime=Ts
  To Workspace18 : ToWorkspace  VariableName=Lambda1  SampleTime=Ts
  To Workspace19 : ToWorkspace  VariableName=Heading_angle_updated1  SampleTime=Ts
      settings: Save2DSignal=2-D array (concatenate along first dimension)
  To Workspace20 : ToWorkspace  VariableName=Lambda3  SampleTime=Ts
  To Workspace21 : ToWorkspace  VariableName=V_OutputError1  SampleTime=Ts
  To Workspace6 : ToWorkspace  VariableName=Y1  SampleTime=Ts
  Unit Delay{18..35} (18 alike) : UnitDelay  SampleTime=Ts
  Visualization1 : Subsystem  TreatAsAtomicUnit=on
      mask Display: disp('Visualization')
  YV_update_Np1 : Subsystem  TreatAsAtomicUnit=on
  Zero-Order Hold3 : ZeroOrderHold  SampleTime=Tf
  Zero-Order Hold4 : ZeroOrderHold  SampleTime=Tf
  Zero-Order Hold5 : ZeroOrderHold  SampleTime=Tf
  wires:
  Rate Transition3/1 -> Simulation Interrupt 1/1(Y), Unit Delay28/1, Front Observer2/1(Y), Sum5/1, Sum2/1, Sum1/1, Sum3/1, Final Observer2/3(Y), Middle Observer2/2(Y), Sum16/2, Sum15/1, To Workspace6/1
  Multiport Switch12/1 -> Mpc_block1/6(Xh)
  Demux1/2 -> MATLAB Function1/1(u)
  Front Observer2/1(yhat) -> Multiport Switch11/2, Sum16/1
  Controllers1/1(Controller) -> Passenger Vehicle1/3(Cntrl)
  Cso2/1 -> Sum1/2
  Front_simulator1/1(Velocity) -> Unit Delay21/1, Mux9/1
  Mux5/1 -> Rate Transition3/1
  Passenger Vehicle1/3(yaw) -> Mux6/3, Mux5/2  "Heading angle  s"
  Sum1/1 -> Multiport Switch9/2
  Front_simulator1/9(OutputError) -> Subsystem2/8(FrontOutputError)
  Unit Delay35/1 -> Final_simulator1/5(udelayMiddle)
  Final_simulator1/11(lambda) -> Multiport Switch2/4
  Sum15/1 -> Multiport Switch8/3
  Unit Delay18/1 -> Final Observer2/6(r(k-1)), Middle Observer2/6(r(k-1))
  Front_simulator1/8(Ldterm) -> Subsystem2/7(FrontLdterm)
  Unit Delay28/1 -> Demux6/1, Demux7/1  "Y_delay"
  Final_simulator1/8(Ldterm) -> Subsystem2/24(FinalLdterm)
  Middle_simulator1/2(Heading_angle) -> Unit Delay26/1, Mux8/2
  Longitudinal Driver1/1(Driver) -> Passenger Vehicle1/2(Steer), Controllers1/1(Pedals), Visualization1/1(Cntrl)
  Final Observer2/3(u_delay) -> H_Final1/1
  Final_simulator1/10(yhat) -> Subsystem2/22(FinalYhat)
  Mpc_block1/1(U) -> Final Observer2/2(U), Middle Observer2/1(U), Front Observer2/2(U), To Workspace15/1, Demux1/1
  Middle_simulator1/7(SyetemError) -> Subsystem2/15(MiddleSystemError)
  Mux8/1 -> Subsystem2/10(MiddleY)
  Mpc_block1/3(Lambda) -> To Workspace18/1
  Middle_simulator1/3(U) -> Unit Delay35/1, Subsystem2/11(MiddleU)
  Final_simulator1/6(Vup) -> Subsystem2/26(FinalVelocityupdate)
  Mux6/1 -> Rate Transition4/1
  Front_simulator1/3(U) -> Subsystem2/2(FrontU), Unit Delay23/1
  Unit Delay33/1 -> Final_simulator1/3(r(k)Middle), Unit Delay34/1
  From Workspace9/1 -> Mpc_block1/2(Rs_V)
  Front_simulator1/10(yhat) -> Subsystem2/9(FrontYhat)
  From Workspace7/1 -> Final_simulator1/1(Rs_V), Middle_simulator1/1(Rs_V), Front_simulator1/1(Rs_V)
  Sum17/1 -> Cso2/1
  Final Observer2/2(xhat_delay) -> G_Final1/1
  Ho2/1 -> Sum18/2
  YV_update_Np1/1(Velocity) -> To Workspace16/1, Mpc_block1/4(Vup)
  Middle_simulator_ operating_time1/1(state) -> Middle_simulator1/Enable
  H_Final1/1 -> Sum4/2
  From Workspace8/1 -> Middle Observer2/3(Rs), Final Observer2/4(Rs), Mpc_block1/1(Rs)
  From Workspace13/1 -> Middle Observer2/10(Tsim), Unit Delay30/1, Final Observer2/11(Tsim)
  Unit Delay24/1 -> Final_simulator1/10(LastT_sim), Middle_simulator1/10(LastT_sim)
  Front_simulator1/11(r(k+1)Front) -> Unit Delay31/1
  From Workspace12/1 -> Final_simulator1/2(Rs), Middle_simulator1/2(Rs)
  Sum4/1 -> C_Final1/1
  Middle_simulator1/5(Rs_heading_angle) -> Subsystem2/13(MiddleHeadingupdate)
  Unit Delay20/1 -> Middle_simulator1/6(PositionfromFront)
  Middle_simulator1/9(OutputError) -> Subsystem2/17(MiddleOutputError)
  Unit Delay31/1 -> Middle_simulator1/3(r(k)Front), Unit Delay32/1
  Middle_simulator1/10(yhat) -> Subsystem2/18(MiddleYhat)
  Unit Delay23/1 -> Middle_simulator1/5(udelayFront)
  YV_update_Np1/2(Heading angle) -> To Workspace19/1, Mpc_block1/5(Rs_heading_angle)
  Unit Delay25/1 -> Final_simulator1/7(VelocitiesfromMiddle)
  Demux7/2 -> Middle Observer2/9(Initial HeadingAngles)
  Front_simulator1/5(Rs_heading_angle) -> Subsystem2/4(FrontHeadingupdate)
  Front_simulator1/6(Vup) -> Subsystem2/5(FrontVelocityupdate)
  Passenger Vehicle1/4(XY) -> Mux6/1, To Workspace17/1, Rate Transition5/1
  Unit Delay22/1 -> Middle_simulator1/8(HeadingAnglesfromFront)
  Final Observer2/1(yhat) -> Sum3/2, Multiport Switch11/4
  Unit Delay21/1 -> Middle_simulator1/7(VelocitiesfromFront)
  MATLAB Function1/2(Br) -> Zero-Order Hold5/1
  Front_simulator1/12(lambda) -> Multiport Switch2/2
  From Workspace10/1 -> Mpc_block1/3(Rs_Y)
  Front_simulator1/4(Position) -> Subsystem2/3(FrontPosition), Unit Delay20/1
  Unit Delay29/1 -> Middle Observer2/4(Initial position), Final Observer2/8(Initial position)
  Middle_simulator1/4(PositionfromMiddle) -> Unit Delay27/1, Subsystem2/12(MiddlePosition)
  Unit Delay30/1 -> Final Observer2/12(LastTsim), Middle Observer2/11(LastTsim)
  Mux7/1 -> Subsystem2/20(FinalY)
  Mpc_block1/2(Ref) -> Unit Delay19/1  "r(k+1)"
  Unit Delay27/1 -> Final_simulator1/6(PositionfromMiddle)
  Observer_state1/1(state) -> Front Observer2/Enable
  Final Observer2/4(xhat) -> Multiport Switch12/4
  Final_simulator1/1(Velocity) -> Mux7/1
  Demux6/2 -> Final Observer2/10(Initial HeadingAngles)
  Unit Delay19/1 -> Final Observer2/7(r(k)), Middle Observer2/7(r(k)), Unit Delay18/1
  Final_simulator1/9(OutputError) -> Subsystem2/21(FinalOutputError)
  Final_simulator1/5(Rs_heading_angle) -> Subsystem2/27(FinalHeadingupdate)
  Multiport Switch2/1 -> To Workspace20/1
  Front_simulator_ operating_time1/1(state) -> Front_simulator1/Enable
  Multiport Switch9/1 -> Lsd2/1, Ld2/1, Ld_Final1/1, To Workspace13/1
  Middle Observer2/1(yhat) -> Multiport Switch11/3, Sum15/2
  From Workspace11/1 -> Unit Delay24/1, Final_simulator1/9(T_sim), Middle_simulator1/9(T_sim)
  Gso2/1 -> Sum17/1
  Middle Observer2/4(xhat) -> Multiport Switch12/3
  Final_simulator1/2(Heading_angle) -> Mux7/2
  Select_model1/1(Select) -> Multiport Switch11/1, Multiport Switch10/1, Multiport Switch9/1, Multiport Switch8/1, Mpc_block1/7(Select), Multiport Switch12/1
  Final_simulator1/3(U) -> Subsystem2/19(FinalU)
  Unit Delay26/1 -> Final_simulator1/8(HeadingAnglesfromMiddle)
  Passenger Vehicle1/1(VehFdbk) -> Controllers1/2(VehFdbk), Visualization1/2(VehFdbk)
  Middle_simulator1/1(Velocity) -> Unit Delay25/1, Mux8/1
  Demux5/2 -> YV_update_Np1/2(Velocity_sim)
  Dataselect1/1(DS) -> Multiport Switch2/1
  Demux6/1 -> Final Observer2/9(Initial Velocities)
  G_Final1/1 -> Sum4/1
  Middle_simulator1/8(Ldterm) -> Subsystem2/16(MiddleLdterm)
  Unit Delay34/1 -> Final_simulator1/4(r(k-1)Middle)
  Sum3/1 -> Multiport Switch8/4
  Passenger Vehicle1/2(Velocity) -> Mux6/2, Mux5/1  "Velocity"
  Sum18/1 -> Co2/1
  Sum16/1 -> Multiport Switch8/2
  Rate Transition4/1 -> Demux5/1
  Mux9/1 -> Subsystem2/1(FrontY)
  Middle_simulator1/6(Vup) -> Subsystem2/14(MiddleVelocityupdate)
  Zero-Order Hold3/1 -> Longitudinal Driver1/1(In1)  "Steer"
  Multiport Switch10/1 -> To Workspace14/1
  Sum5/1 -> Multiport Switch9/4
  Environment1/1(Env) -> Passenger Vehicle1/1(Env)
  MATLAB Function1/1(Ac) -> Zero-Order Hold4/1
  Demux1/1 -> Zero-Order Hold3/1
  Zero-Order Hold5/1 -> Longitudinal Driver1/3(In3)  "Brake"
  Middle_simulator1/12(lambda) -> Multiport Switch2/3
  Demux7/1 -> Middle Observer2/8(Initial Velocities)
  Final_simulator_ operating_time1/1(state) -> Final_simulator1/Enable
  Front_simulator1/7(SyetemError) -> Subsystem2/6(FrontSystemError)
  Front Observer2/2(xhat_delay) -> Gso2/1
  Unit Delay32/1 -> Middle_simulator1/4(r(k-1)Front)
  Lsd2/1 -> Multiport Switch10/2
  Demux5/3 -> YV_update_Np1/3(Heading_sim)
  Front Observer2/3(u_delay) -> Middle Observer2/5(U_delay), Hso2/1
  Final_simulator1/4(PositionfromFinal) -> Subsystem2/25(FinalPosition)
  Middle_simulator1/11(r(k+1)Middle) -> Unit Delay33/1
  Final_simulator1/7(SyetemError) -> Subsystem2/23(FinalSystemError)
  Middle Observer2/3(u_delay) -> Final Observer2/5(U_delay), Ho2/1
  C_Final1/1 -> Sum5/2
  Observer_state3/1(state) -> Final Observer2/Enable
  Zero-Order Hold4/1 -> Longitudinal Driver1/2(In2)  "Acceleration"
  Front Observer2/4(xhat) -> Multiport Switch12/2
  Go2/1 -> Sum18/1
  Sum2/1 -> Multiport Switch9/3
  Multiport Switch11/1 -> To Workspace12/1
  Multiport Switch8/1 -> To Workspace21/1
  Observer_state2/1(state) -> Middle Observer2/Enable
  Demux5/1 -> YV_update_Np1/1(XY_sim)
  Front_simulator1/2(Heading_angle) -> Mux9/2, Unit Delay22/1
  Rate Transition5/1 -> Unit Delay29/1
  Ld2/1 -> Multiport Switch10/3
  Middle Observer2/2(xhat_delay) -> Go2/1
  Ld_Final1/1 -> Multiport Switch10/4
  Hso2/1 -> Sum17/2
  Co2/1 -> Sum2/2
  In1/1 -> Final Observer2/1(Final_switch)

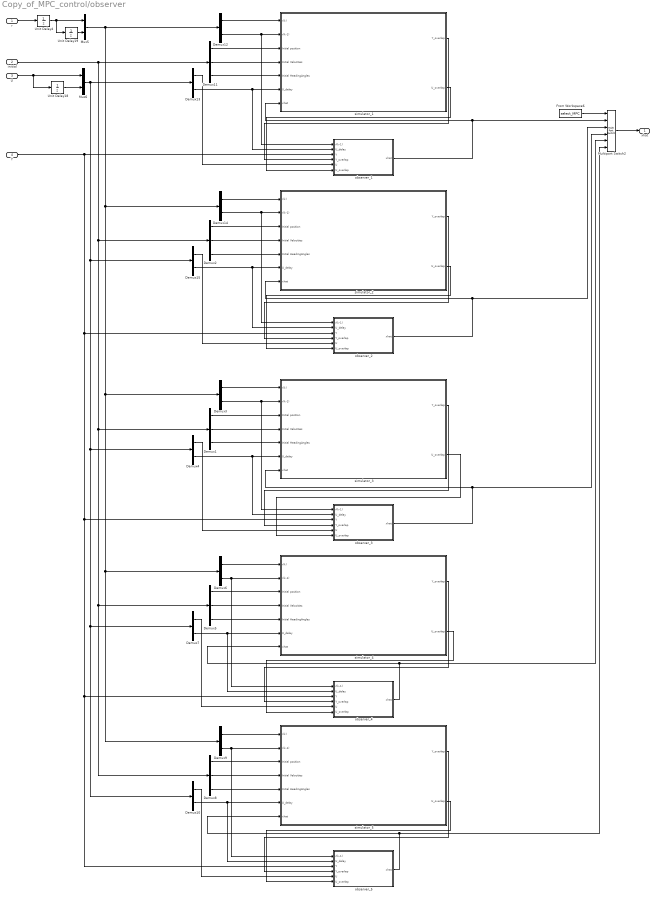
== system Copy_of_MPC_control/observer ==
  r : Inport
  initial : Inport  Port=2
  U : Inport  Port=3
  Y : Inport  Port=4
  Demux{1..2,5,8,11} (5 alike) : Demux  Outputs=3
  Demux{3..4,6..7,9..10,12..15} (10 alike) : Demux  Outputs=2
  From Workspace6 : FromWorkspace  VariableName=select_MPC  SampleTime=Ts
  Multiport Switch2 : MultiPortSwitch  Inputs=5
  Mux5 : Mux  Inputs=2
  Mux6 : Mux  Inputs=2
  Unit Delay18 : UnitDelay  SampleTime=Ts
  Unit Delay19 : UnitDelay  InitialCondition=ro  SampleTime=Ts
  Unit Delay4 : UnitDelay  InitialCondition=ro  SampleTime=Ts
  observer_1 : Subsystem
  observer_2 : Subsystem
  observer_3 : Subsystem
  observer_4 : Subsystem
  observer_5 : Subsystem
  simulator_1 : Subsystem
  simulator_2 : Subsystem
  simulator_3 : Subsystem
  simulator_4 : Subsystem
  simulator_5 : Subsystem
  xhat : Outport
  wires:
  observer_4/1(xhat) -> Multiport Switch2/5, simulator_4/7(xhat)
  Demux6/1 -> simulator_4/1(r(k))
  observer_3/1(xhat) -> Multiport Switch2/4, simulator_3/7(xhat)
  Demux8/1 -> simulator_5/3(Initial position)
  Demux1/1 -> simulator_3/3(Initial position)
  Demux4/2 -> observer_3/2(U_delay), simulator_3/6(U_delay)
  Demux13/1 -> observer_1/5(U)
  simulator_4/2(U_overlap) -> observer_4/6(U_overlap)
  simulator_4/1(Y_overlap) -> observer_4/4(Y_overlap)
  Demux5/3 -> simulator_4/5(Initial HeadingAngles)
  Demux3/2 -> observer_3/1(r(k-1)), simulator_3/2(r(k-1))
  Demux8/2 -> simulator_5/4(Initial Velocities)
  Demux7/2 -> observer_4/2(U_delay), simulator_4/6(U_delay)
  simulator_5/1(Y_overlap) -> observer_5/4(Y_overlap)
  Demux6/2 -> observer_4/1(r(k-1)), simulator_4/2(r(k-1))
  observer_5/1(xhat) -> Multiport Switch2/6, simulator_5/7(xhat)
  Demux9/2 -> observer_5/1(r(k-1)), simulator_5/2(r(k-1))
  Demux10/2 -> observer_5/2(U_delay), simulator_5/6(U_delay)
  Demux11/1 -> simulator_1/3(Initial position)
  Demux13/2 -> observer_1/2(U_delay), simulator_1/6(U_delay)
  Demux5/2 -> simulator_4/4(Initial Velocities)
  Demux9/1 -> simulator_5/1(r(k))
  simulator_3/1(Y_overlap) -> observer_3/4(Y_overlap)
  Demux1/2 -> simulator_3/4(Initial Velocities)
  simulator_3/2(U_overlap) -> observer_3/6(U_overlap)
  Demux12/2 -> observer_1/1(r(k-1)), simulator_1/2(r(k-1))
  Demux10/1 -> observer_5/5(U)
  Demux8/3 -> simulator_5/5(Initial HeadingAngles)
  Demux7/1 -> observer_4/5(U)
  simulator_5/2(U_overlap) -> observer_5/6(U_overlap)
  Demux11/2 -> simulator_1/4(Initial Velocities)
  Demux5/1 -> simulator_4/3(Initial position)
  simulator_1/2(U_overlap) -> observer_1/6(U_overlap)
  Demux4/1 -> observer_3/5(U)
  Demux3/1 -> simulator_3/1(r(k))
  Demux12/1 -> simulator_1/1(r(k))
  Demux1/3 -> simulator_3/5(Initial HeadingAngles)
  simulator_1/1(Y_overlap) -> observer_1/4(Y_overlap)
  observer_1/1(xhat) -> Multiport Switch2/2, simulator_1/7(xhat)
  Demux11/3 -> simulator_1/5(Initial HeadingAngles)
  From Workspace6/1 -> Multiport Switch2/1
  Multiport Switch2/1 -> xhat/1
  r/1 -> Unit Delay4/1
  Unit Delay4/1 -> Mux5/1, Unit Delay19/1
  Unit Delay19/1 -> Mux5/2
  Unit Delay18/1 -> Mux6/2
  U/1 -> Mux6/1, Unit Delay18/1
  simulator_2/2(U_overlap) -> observer_2/6(U_overlap)
  simulator_2/1(Y_overlap) -> observer_2/4(Y_overlap)
  Demux2/3 -> simulator_2/5(Initial HeadingAngles)
  Demux2/2 -> simulator_2/4(Initial Velocities)
  Demux14/1 -> simulator_2/1(r(k))
  Y/1 -> observer_2/3(Y), observer_3/3(Y), observer_5/3(Y), observer_4/3(Y), observer_1/3(Y)
  Mux6/1 -> Demux15/1, Demux4/1, Demux7/1, Demux10/1, Demux13/1
  initial/1 -> Demux11/1, Demux2/1, Demux1/1, Demux5/1, Demux8/1
  Demux15/2 -> observer_2/2(U_delay), simulator_2/6(U_delay)
  Mux5/1 -> Demux14/1, Demux3/1, Demux6/1, Demux9/1, Demux12/1
  observer_2/1(xhat) -> Multiport Switch2/3, simulator_2/7(xhat)
  Demux2/1 -> simulator_2/3(Initial position)
  Demux14/2 -> observer_2/1(r(k-1)), simulator_2/2(r(k-1))
  Demux15/1 -> observer_2/5(U)

== system Copy_of_MPC_control/observer for ID ==
  U : Inport
  Udelay : Inport  Port=2
  Y : Inport  Port=3
  r(k) : Inport  Port=4
  ID_interval : Inport  Port=5
  Delay : Delay  DelayLength=1  InitialConditionSource=Input port  InitialCondition=0  ExternalReset=Rising  SampleTime=Ts
      settings: InputPortMap=u0,r5,p4
  Delay2 : Delay  DelayLength=1  InitialConditionSource=Input port  InitialCondition=0  ExternalReset=Rising  SampleTime=Ts
      settings: InputPortMap=u0,r5,p4
  Gd : Gain  Gain=Gd  Multiplication=Matrix(K*u) (u vector)
  Hd : Gain  Gain=Hd  Multiplication=Matrix(K*u) (u vector)
  Ld : Gain  Gain=Ld  Multiplication=Matrix(K*u) (u vector)
  Ld* : Gain  Gain=Ld  Multiplication=Matrix(K*u) (u vector)
  Sum4 : Sum  Inputs=+++
  xhat : Outport
  wires:
  Hd/1 -> Sum4/2
  Ld*/1 -> Sum4/1
  Gd/1 -> Sum4/3
  Ld/1 -> Delay/3
  Sum4/1 -> Delay/1, xhat/1  "xhat"
  Delay/1 -> Gd/1
  r(k)/1 -> Ld/1
  Y/1 -> Ld*/1
  Delay2/1 -> Hd/1
  U/1 -> Delay2/1
  ID_interval/1 -> Delay2/2, Delay/2
  Udelay/1 -> Delay2/3

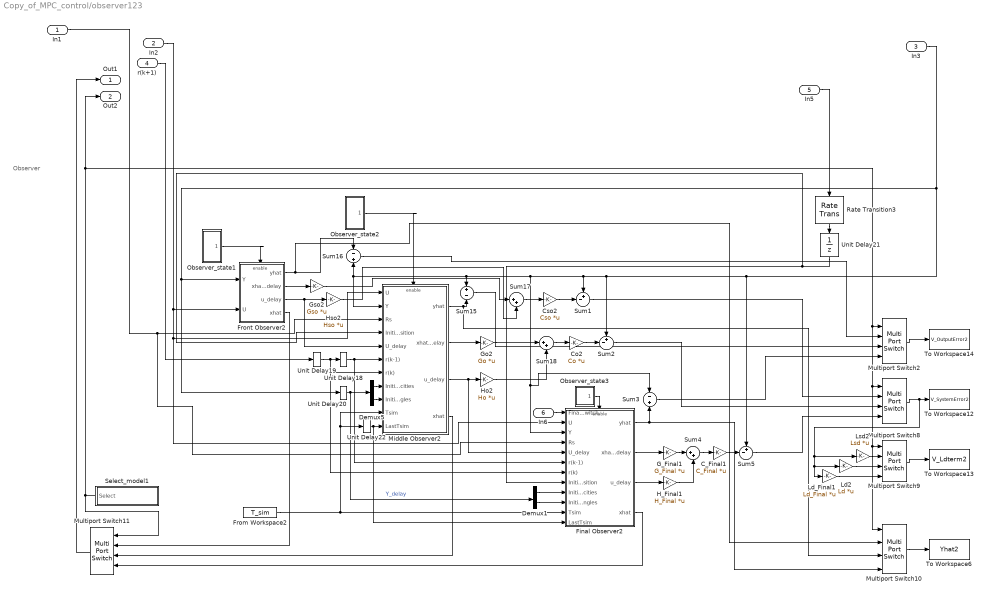
== system Copy_of_MPC_control/observer123 ==
  note: Observer
  In1 : Inport
  In2 : Inport  Port=2
  In3 : Inport  Port=3
  r(k+1) : Inport  Port=4
  In5 : Inport  Port=5
  In6 : Inport  Port=6
  C_Final1 : Gain  Gain=C_Final  Multiplication=Matrix(K*u) (u vector)
  Co2 : Gain  Gain=Co  Multiplication=Matrix(K*u) (u vector)
  Cso2 : Gain  Gain=Cso  Multiplication=Matrix(K*u) (u vector)
  Demux1 : Demux  Outputs=2
  Demux5 : Demux  Outputs=2
  Final Observer2 : Subsystem
  From Workspace2 : FromWorkspace  VariableName=T_sim  SampleTime=Ts
  Front Observer2 : Subsystem
  G_Final1 : Gain  Gain=G_Final  Multiplication=Matrix(K*u) (u vector)
  Go2 : Gain  Gain=Go  Multiplication=Matrix(K*u) (u vector)
  Gso2 : Gain  Gain=Gso  Multiplication=Matrix(K*u) (u vector)
  H_Final1 : Gain  Gain=H_Final  Multiplication=Matrix(K*u) (u vector)
  Ho2 : Gain  Gain=Ho  Multiplication=Matrix(K*u) (u vector)
  Hso2 : Gain  Gain=Hso  Multiplication=Matrix(K*u) (u vector)
  Ld2 : Gain  Gain=Ld  Multiplication=Matrix(K*u) (u vector)
  Ld_Final1 : Gain  Gain=Ld_Final  Multiplication=Matrix(K*u) (u vector)
  Lsd2 : Gain  Gain=Lsd  Multiplication=Matrix(K*u) (u vector)
  Middle Observer2 : Subsystem
  Multiport Switch{2,8..11} (5 alike) : MultiPortSwitch
  Observer_state1 : Subsystem
  Observer_state2 : Subsystem
  Observer_state3 : Subsystem
  Rate Transition3 : RateTransition  OutPortSampleTime=Ts
  Select_model1 : Subsystem
  Sum1 : Sum  Inputs=+-|
  Sum15 : Sum  Inputs=+-
  Sum16 : Sum  Inputs=-+
  Sum17 : Sum  Inputs=|++
  Sum18 : Sum  Inputs=|++
  Sum2 : Sum  Inputs=+-|
  Sum3 : Sum  Inputs=-+
  Sum4 : Sum  Inputs=|++
  Sum5 : Sum  Inputs=+-|
  To Workspace12 : ToWorkspace  VariableName=V_SystemError2  SampleTime=Ts
  To Workspace13 : ToWorkspace  VariableName=V_Ldterm2  SampleTime=Ts
  To Workspace14 : ToWorkspace  VariableName=V_OutputError2  SampleTime=Ts
  To Workspace6 : ToWorkspace  VariableName=Yhat2  SampleTime=Ts
  Unit Delay{18..22} (5 alike) : UnitDelay  SampleTime=Ts
  Out1 : Outport
  Out2 : Outport  Port=2
  wires:
  Cso2/1 -> Sum1/2
  In3/1 -> Unit Delay20/1, Front Observer2/1(Y), Sum5/1, Sum2/1, Sum1/1, Sum3/1, Final Observer2/3(Y), Middle Observer2/2(Y), Sum16/2, Sum15/1
  Sum4/1 -> C_Final1/1
  Sum5/1 -> Multiport Switch8/4
  Multiport Switch8/1 -> Lsd2/1, Ld2/1, Ld_Final1/1, To Workspace12/1
  From Workspace2/1 -> Middle Observer2/10(Tsim), Unit Delay22/1, Final Observer2/11(Tsim)
  Sum18/1 -> Co2/1
  Front Observer2/3(u_delay) -> Middle Observer2/5(U_delay), Hso2/1
  Sum15/1 -> Multiport Switch2/3
  Final Observer2/1(yhat) -> Sum3/2, Multiport Switch10/4
  In2/1 -> Final Observer2/2(U), Middle Observer2/1(U), Front Observer2/2(U)
  Ho2/1 -> Sum18/2
  Hso2/1 -> Sum17/2
  Unit Delay20/1 -> Demux1/1, Demux5/1  "Y_delay"
  Unit Delay22/1 -> Final Observer2/12(LastTsim), Middle Observer2/11(LastTsim)
  Middle Observer2/4(xhat) -> Multiport Switch11/3
  In1/1 -> Middle Observer2/3(Rs), Final Observer2/4(Rs)
  Unit Delay21/1 -> Middle Observer2/4(Initial position), Final Observer2/8(Initial position)
  Front Observer2/1(yhat) -> Multiport Switch10/2, Sum16/1
  Final Observer2/3(u_delay) -> H_Final1/1
  Final Observer2/2(xhat_delay) -> G_Final1/1
  Gso2/1 -> Sum17/1
  Front Observer2/4(xhat) -> Multiport Switch11/2
  Go2/1 -> Sum18/1
  Demux5/1 -> Middle Observer2/8(Initial Velocities)
  Final Observer2/4(xhat) -> Multiport Switch11/4
  Multiport Switch11/1 -> Out1/1
  Observer_state3/1(state) -> Final Observer2/Enable
  Ld_Final1/1 -> Multiport Switch9/4
  Demux1/2 -> Final Observer2/10(Initial HeadingAngles)
  C_Final1/1 -> Sum5/2
  Sum2/1 -> Multiport Switch8/3
  Sum1/1 -> Multiport Switch8/2
  Middle Observer2/2(xhat_delay) -> Go2/1
  Observer_state2/1(state) -> Middle Observer2/Enable
  Sum16/1 -> Multiport Switch2/2
  In6/1 -> Final Observer2/1(Final_switch)
  G_Final1/1 -> Sum4/1
  Middle Observer2/1(yhat) -> Multiport Switch10/3, Sum15/2
  H_Final1/1 -> Sum4/2
  Rate Transition3/1 -> Unit Delay21/1
  Observer_state1/1(state) -> Front Observer2/Enable
  Demux5/2 -> Middle Observer2/9(Initial HeadingAngles)
  Multiport Switch2/1 -> To Workspace14/1
  Select_model1/1(Select) -> Out2/1, Multiport Switch10/1, Multiport Switch9/1, Multiport Switch8/1, Multiport Switch2/1, Multiport Switch11/1
  Lsd2/1 -> Multiport Switch9/2
  Front Observer2/2(xhat_delay) -> Gso2/1
  Sum3/1 -> Multiport Switch2/4
  Middle Observer2/3(u_delay) -> Final Observer2/5(U_delay), Ho2/1
  Unit Delay19/1 -> Final Observer2/7(r(k)), Middle Observer2/7(r(k)), Unit Delay18/1
  Multiport Switch9/1 -> To Workspace13/1
  Co2/1 -> Sum2/2
  Ld2/1 -> Multiport Switch9/3
  Sum17/1 -> Cso2/1
  Demux1/1 -> Final Observer2/9(Initial Velocities)
  Unit Delay18/1 -> Final Observer2/6(r(k-1)), Middle Observer2/6(r(k-1))
  Multiport Switch10/1 -> To Workspace6/1
  r(k+1)/1 -> Unit Delay19/1
  In5/1 -> Rate Transition3/1

== system Copy_of_MPC_control/plot_reference ==
  Clock : Clock
  Constant : Constant  Value=XYplot  SampleTime=Ts
  MATLAB Function1 : MATLAB Function  TreatAsAtomicUnit=on
  wires:
  Clock/1 -> MATLAB Function1/2(Tsim)
  Constant/1 -> MATLAB Function1/1(XYplot)

== system Copy_of_MPC_control/stop ==
  Y : Inport
  U : Inport  Port=2
  Abs{,1..3} (4 alike) : Abs
  Constant : Constant
  Constant1 : Constant  Value=0
  Fcn{,1,4..5} (4 alike) : Fcn  Expr=u(1)
  Fcn{2..3,6..7} (4 alike) : Fcn  Expr=u(2)
  From Workspace : FromWorkspace  VariableName=U_ref  SampleTime=Ts
  From Workspace1 : FromWorkspace  VariableName=Y_ref  SampleTime=Ts
  From Workspace2 : FromWorkspace  VariableName=Y_ref  SampleTime=Ts
  From Workspace3 : FromWorkspace  VariableName=U_ref  SampleTime=Ts
  Stop Simulation : Stop
  Sum{1..4} (4 alike) : Sum  Inputs=|+-
  Sum5 : Sum  Inputs=|++++
  Switch : Switch  Threshold=0.03
  To Workspace : ToWorkspace  VariableName=total_error  SampleTime=Ts
  wires:
  From Workspace1/1 -> Fcn1/1
  Fcn/1 -> Sum4/2
  Fcn1/1 -> Sum4/1
  Sum4/1 -> Abs/1
  Fcn3/1 -> Sum1/1
  Sum1/1 -> Abs1/1
  Y/1 -> Fcn/1, Fcn2/1
  Fcn2/1 -> Sum1/2
  From Workspace2/1 -> Fcn3/1
  Fcn4/1 -> Sum2/2
  Sum2/1 -> Abs2/1
  Fcn5/1 -> Sum2/1
  From Workspace/1 -> Fcn5/1
  U/1 -> Fcn4/1, Fcn6/1
  Sum3/1 -> Abs3/1
  Fcn7/1 -> Sum3/1
  Fcn6/1 -> Sum3/2
  From Workspace3/1 -> Fcn7/1
  Constant/1 -> Switch/1
  Constant1/1 -> Switch/3
  Switch/1 -> Stop Simulation/1
  Sum5/1 -> Switch/2, To Workspace/1
  Abs1/1 -> Sum5/2
  Abs2/1 -> Sum5/3
